simulink model "Kangaroo_Island_Microgrid1"  (R2025b)
settings: Solver=VariableStepAuto  StartTime=0.0  StopTime=10.0  RelTol=1e-3
model workspace (MAT data in the model file):
  base_load = 50
  battery_capacity = 500
  battery_efficiency = 0.9
  battery_initial_soc = 0.5
  battery_max_soc = 0.95
  battery_min_soc = 0.2
  battery_power = 150
  dt = 1
  grid_export_price = 0.1
  grid_import_cost = 0.35
  peak_load = 120
  pv_capacity = 200
  pv_derating = 0.85
  pv_efficiency = 0.18
  sim_hours = 8760
  wt_capacity = 150
  wt_cut_in = 3
  wt_cut_out = 25
  wt_rated_speed = 12

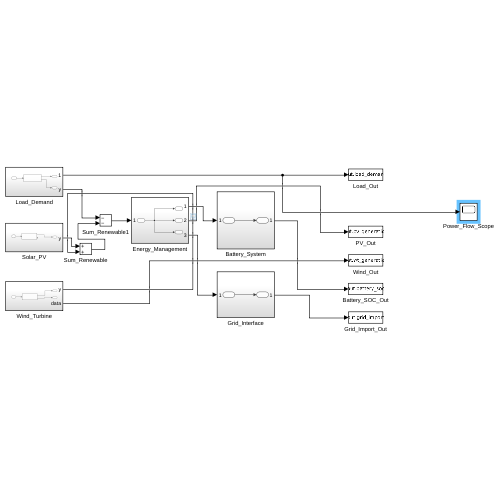
[thumbnail: Simulink's stored preview of the top-level diagram]
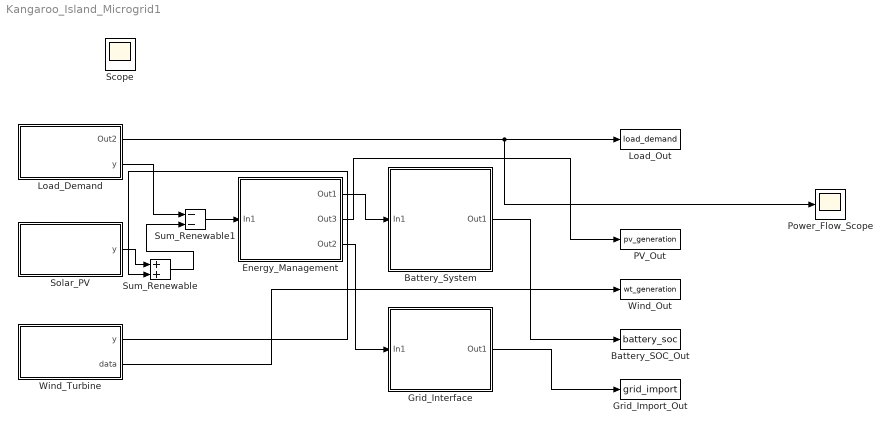
== system Kangaroo_Island_Microgrid1 ==
  Battery_SOC_Out : ToWorkspace  VariableName=battery_soc  SaveFormat=Timeseries  SampleTime=-1
  Battery_System : Subsystem
  Energy_Management : Subsystem
  Grid_Import_Out : ToWorkspace  VariableName=grid_import  SaveFormat=Timeseries  SampleTime=-1
  Grid_Interface : Subsystem
  Load_Demand : Subsystem
  Load_Out : ToWorkspace  VariableName=load_demand  SaveFormat=Timeseries  SampleTime=-1
  PV_Out : ToWorkspace  VariableName=pv_generation  SaveFormat=Timeseries  SampleTime=-1
  Power_Flow_Scope : Scope
      settings: ActiveDisplayYMinimum=-1  ActiveDisplayYMaximum=1
  Solar_PV : Subsystem
  Sum_Renewable : Sum
  Sum_Renewable1 : Sum  Inputs=--
  Wind_Out : ToWorkspace  VariableName=wt_generation  SaveFormat=Timeseries  SampleTime=-1
  Wind_Turbine : Subsystem
  Scope : Scope
  wires:
  Load_Demand/2(y) -> Sum_Renewable1/1
  Solar_PV/1(y) -> Sum_Renewable/1
  Wind_Turbine/1(y) -> Sum_Renewable/2
  Sum_Renewable/1 -> Sum_Renewable1/2
  Sum_Renewable1/1 -> Energy_Management/1(In1)
  Energy_Management/1(Out1) -> Battery_System/1(In1)
  Energy_Management/3(Out2) -> Grid_Interface/1(In1)
  Load_Demand/1(Out2) -> Power_Flow_Scope/1, Load_Out/1
  Energy_Management/2(Out3) -> PV_Out/1
  Grid_Interface/1(Out1) -> Grid_Import_Out/1
  Battery_System/1(Out1) -> Battery_SOC_Out/1
  Wind_Turbine/2(data) -> Wind_Out/1

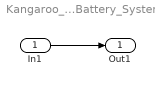
== system Kangaroo_Island_Microgrid1/Battery_System ==
  In1 : Inport
  Out1 : Outport
  wires:
  In1/1 -> Out1/1

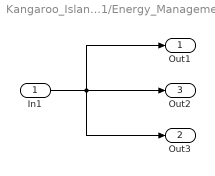
== system Kangaroo_Island_Microgrid1/Energy_Management ==
  In1 : Inport
  Out1 : Outport
  Out3 : Outport  Port=2
  Out2 : Outport  Port=3
  wires:
  In1/1 -> Out3/1, Out1/1, Out2/1

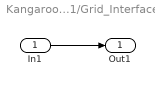
== system Kangaroo_Island_Microgrid1/Grid_Interface ==
  In1 : Inport
  Out1 : Outport
  wires:
  In1/1 -> Out1/1

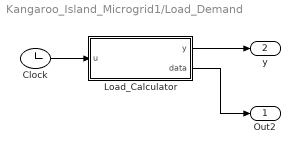
== system Kangaroo_Island_Microgrid1/Load_Demand ==
  Clock : Clock
  Load_Calculator : MATLAB Function  TreatAsAtomicUnit=on
  Out2 : Outport
  y : Outport  Port=2
  wires:
  Clock/1 -> Load_Calculator/1(u)
  Load_Calculator/1(y) -> y/1
  Load_Calculator/2(data) -> Out2/1

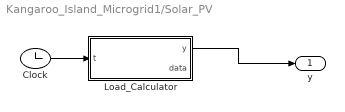
== system Kangaroo_Island_Microgrid1/Solar_PV ==
  Clock : Clock
  Load_Calculator : MATLAB Function  TreatAsAtomicUnit=on
  y : Outport
  wires:
  Clock/1 -> Load_Calculator/1(t)
  Load_Calculator/1(y) -> y/1

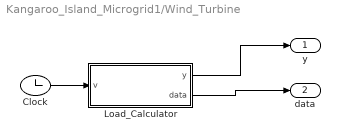
== system Kangaroo_Island_Microgrid1/Wind_Turbine ==
  Clock : Clock
  Load_Calculator : MATLAB Function  TreatAsAtomicUnit=on
  y : Outport
  data : Outport  Port=2
  wires:
  Clock/1 -> Load_Calculator/1(v)
  Load_Calculator/1(y) -> y/1
  Load_Calculator/2(data) -> data/1

== matlab function Kangaroo_Island_Microgrid1/Load_Demand/Load_Calculator ==
  data: u input; y output; data output
function [y, data] = fcn(u)
    y = 2*u;
    data = y;
end

== matlab function Kangaroo_Island_Microgrid1/Wind_Turbine/Load_Calculator ==
  data: v input; y output; data output
function [y, data] = wind_turbine(v)
% Calculate wind turbine power output
% Inputs:
%   v - wind speed at current time (m/s)
% Outputs:
%   y - turbine power output at that wind speed (kW)
%   data - optional output, same as y

    % --- Wind turbine parameters ---
    wt_capacity = 150;    % kW rated power
    wt_cut_in = 3;        % m/s
    wt_rated_speed = 12;  % m/s
    wt_cut_out = 25;      % m/s
    
    % --- Power calculation ---
    if v < wt_cut_in || v > wt_cut_out
        y = 0;
    elseif v >= wt_cut_in && v < wt_rated_speed
        y = wt_capacity * ((v^3 - wt_cut_in^3)/(wt_rated_speed^3 - wt_cut_in^3));
    else
        y = wt_capacity;
    end
    
    % Optional data output
    data = y;
end

== matlab function Kangaroo_Island_Microgrid1/Solar_PV/Load_Calculator ==
  data: t input; y output; data output
function [y, data] = solar_PV(t)
% Calculate PV generation for Kangaroo Island microgrid
% Inputs:
%   t - current simulation hour (1..8760)
% Outputs:
%   y - PV generation at hour t (kW)
%   data - optional output, same as y

    % --- PV system parameters ---
    pv_capacity = 200;    % kW
    pv_derating = 0.85;   % derating factor
    
    % --- Determine hour and day ---
    hour_of_day = mod(t-1, 24);      % 0 to 23
    day_of_year = floor((t-1)/24)+1; % 1 to 365
    
    % --- Solar irradiance calculation ---
    if hour_of_day >= 6 && hour_of_day <= 18
        % Peak irradiance at noon
        solar_irr = 800 * sin(pi*(hour_of_day-6)/12); % W/m^2
    else
        solar_irr = 0;
    end
    
    % Seasonal adjustment
    seasonal_factor = 1 + 0.3*sin(2*pi*(day_of_year-80)/365);
    solar_irr = solar_irr * seasonal_factor;
    
    % Optional cloud cover / randomness can be omitted for deterministic simulation
    
    % --- PV generation ---
    y = (solar_irr / 1000) * pv_capacity * pv_derating; % kW
    
    % Optional data output
    data = y;
end
